simulink model "B100A_Inlet"  (R2024a)
settings: Solver=VariableStepAuto  StartTime=0.0  StopTime=10.0  RelTol=1e-3
undefined symbols (not defined in the file): CCS1, CCS2, GB, T, Type1, Type2
libraries: simulink x2
settings Model: DataDictionary=EVSE_Root_dict.sldd  Creator=jh2beauty  LastModifiedBy=jh2beauty

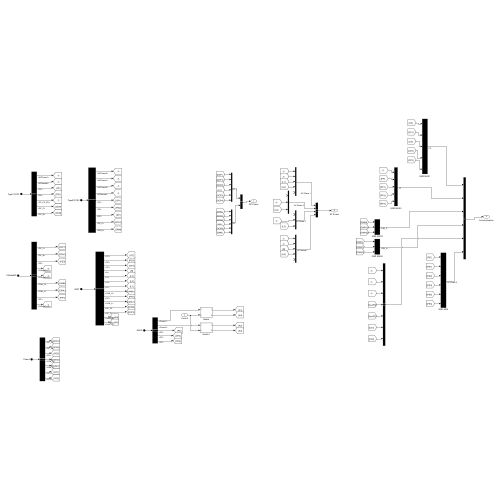
[thumbnail: Simulink's stored preview of the top-level diagram]
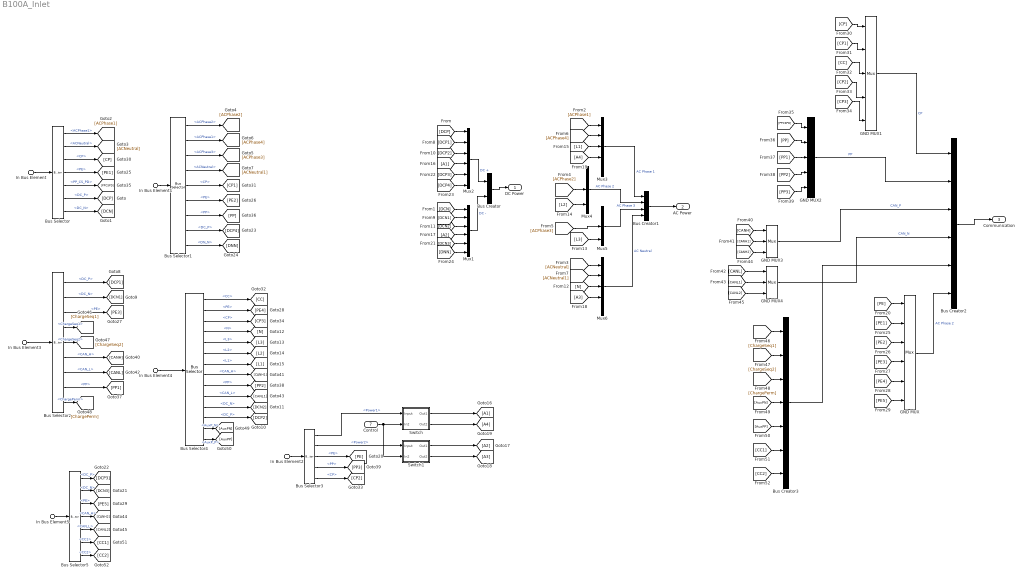
== system B100A_Inlet ==
  In Bus Element : Inport  PortName=Type1/CCS1
  In Bus Element1 : Inport  Port=2  PortName=Type2/CCS2
  In Bus Element2 : Inport  Port=3  PortName=NACS
  In Bus Element3 : Inport  Port=4  PortName=CHAdeMO
  In Bus Element4 : Inport  Port=5  PortName=GB/T
  In Bus Element5 : Inport  Port=6  PortName=ChaoJi
  Control : Inport  Port=7
  Bus Creator : BusCreator  Inputs=2
  Bus Creator1 : BusCreator  Inputs=4
  Bus Creator2 : BusCreator  Inputs=6
  Bus Creator3 : BusCreator  Inputs=7
  Bus Selector : BusSelector  OutputSignals=ACPhase1,ACNeutral,CP,PE,PP_CS_PD,DC_P,DC_N
  Bus Selector1 : BusSelector  OutputSignals=ACPhase2,ACPhase1,ACPhase3,ACNeutral,CP,PE,PP,DC_P,DN_N
  Bus Selector2 : BusSelector  OutputSignals=DC_P,DC_N,PE,ChargeSeq1,ChargeSeq2,CAN_H,CAN_L,PP,ChargePerm
  Bus Selector3 : BusSelector  OutputSignals=Power1,Power2,PE,PP,CP
  Bus Selector4 : BusSelector  OutputSignals=CC,PE,CP,N,L3,L2,L1,CAN_H,PP,CAN_L,DC_N,DC_P,AuxP_N,AuxP_P
  Bus Selector5 : BusSelector  OutputSignals=DC_P,DC_N,PE,CAN_H,CAN_L,CC1,CC2
  GND MUX : Mux  Inputs=6
  GND MUX1 : Mux  Inputs=5
  GND MUX2 : Mux  Inputs=5
  GND MUX3 : Mux  Inputs=3
  GND MUX4 : Mux  Inputs=3
  Mux1 : Mux  Inputs=6
  Mux2 : Mux  Inputs=6
  Mux3 : Mux  Inputs=5
  Mux4 : Mux  Inputs=3
  Mux5 : Mux  Inputs=3
  Mux6 : Mux  Inputs=5
  Switch : Subsystem
  Switch1 : Subsystem
  DC Power : Outport
  AC Power : Outport  Port=2
  Communication : Outport  Port=3
  wires:
  In Bus Element/1 -> Bus Selector/1
  In Bus Element1/1 -> Bus Selector1/1
  Bus Creator/1 -> DC Power/1
  Bus Creator1/1 -> AC Power/1
  Bus Creator2/1 -> Communication/1
  Mux2/1 -> Bus Creator/1  "DC +"
  Mux1/1 -> Bus Creator/2  "DC -"
  Mux3/1 -> Bus Creator1/1  "AC Phase 1"
  Mux4/1 -> Bus Creator1/2  "AC Phase 2"
  Mux5/1 -> Bus Creator1/3  "AC Phase 3"
  Mux6/1 -> Bus Creator1/4  "AC Neutral"
  In Bus Element3/1 -> Bus Selector2/1
  In Bus Element2/1 -> Bus Selector3/1
  Bus Selector/6 -> [DCP]  "<DC_P>"
  [DCP] -> Mux2/1
  Bus Selector/7 -> [DCN]  "<DC_N>"
  [DCN] -> Mux1/1
  Bus Selector/1 -> [ACPhase1]  "<ACPhase1>"
  [ACPhase1] -> Mux3/1
  Bus Selector/2 -> [ACNeutral]  "<ACNeutral>"
  [ACNeutral] -> Mux6/1
  Bus Selector1/1 -> [ACPhase2]  "<ACPhase2>"
  [ACPhase2] -> Mux4/2
  Bus Selector1/3 -> [ACPhase3]  "<ACPhase3>"
  [ACPhase3] -> Mux5/2
  Bus Selector1/2 -> [ACPhase4]  "<ACPhase1>"
  [ACPhase4] -> Mux3/2
  Bus Selector1/4 -> [ACNeutral1]  "<ACNeutral>"
  [ACNeutral1] -> Mux6/2
  In Bus Element4/1 -> Bus Selector4/1
  In Bus Element5/1 -> Bus Selector5/1
  Bus Selector3/1 -> Switch/1(Input)  "<Power1>"
  Bus Selector3/2 -> Switch1/1(Input)  "<Power2>"
  Bus Selector2/1 -> [DCP1]  "<DC_P>"
  [DCP1] -> Mux2/2
  Bus Selector2/2 -> [DCN1]  "<DC_N>"
  [DCN1] -> Mux1/2
  Bus Selector4/12 -> [DCP2]  "<DC_P>"
  [DCP2] -> Mux2/3
  Bus Selector4/11 -> [DCN2]  "<DC_N>"
  [DCN2] -> Mux1/3
  Bus Selector4/4 -> [N]  "<N>"
  [N] -> Mux6/3
  Bus Selector4/5 -> [L3]  "<L3>"
  [L3] -> Mux5/3
  Bus Selector4/6 -> [L2]  "<L2>"
  [L2] -> Mux4/3
  Bus Selector4/7 -> [L1]  "<L1>"
  [L1] -> Mux3/3
  Switch/1(Out1) -> [A1]
  [A1] -> Mux2/4
  Switch1/1(Out1) -> [A2]
  [A2] -> Mux1/4
  Switch1/2(Out2) -> [A3]
  [A3] -> Mux6/4
  Switch/2(Out2) -> [A4]
  [A4] -> Mux3/4
  Control/1 -> Switch1/2(In2), Switch/2(In2)
  Bus Selector3/3 -> [PE]  "<PE>"
  [PE] -> GND MUX/1
  Bus Selector5/2 -> [DCN3]  "<DC_N>"
  [DCN3] -> Mux1/5
  Bus Selector5/1 -> [DCP3]  "<DC_P>"
  [DCP3] -> Mux2/5
  Bus Selector1/8 -> [DCP4]  "<DC_P>"
  [DCP4] -> Mux2/6
  Bus Selector1/9 -> [DNN]  "<DN_N>"
  [DNN] -> Mux1/6
  Bus Selector/4 -> [PE1]  "<PE>"
  [PE1] -> GND MUX/2
  Bus Selector1/6 -> [PE2]  "<PE>"
  [PE2] -> GND MUX/3
  Bus Selector2/3 -> [PE3]  "<PE>"
  [PE3] -> GND MUX/4
  Bus Selector4/2 -> [PE4]  "<PE>"
  [PE4] -> GND MUX/5
  Bus Selector5/3 -> [PE5]  "<PE>"
  [PE5] -> GND MUX/6
  Bus Selector/3 -> [CP]  "<CP>"
  [CP] -> GND MUX1/1
  Bus Selector1/5 -> [CP1]  "<CP>"
  [CP1] -> GND MUX1/2
  Bus Selector4/1 -> [CC]  "<CC>"
  [CC] -> GND MUX1/3
  Bus Selector3/5 -> [CP2]  "<CP>"
  [CP2] -> GND MUX1/4
  Bus Selector4/3 -> [CP3]  "<CP>"
  [CP3] -> GND MUX1/5
  Bus Selector/5 -> [PPCSPD]  "<PP_CS_PD>"
  [PPCSPD] -> GND MUX2/1
  Bus Selector1/7 -> [PP]  "<PP>"
  [PP] -> GND MUX2/2
  Bus Selector2/8 -> [PP1]  "<PP>"
  [PP1] -> GND MUX2/3
  Bus Selector4/9 -> [PP2]  "<PP>"
  [PP2] -> GND MUX2/4
  Bus Selector3/4 -> [PP3]  "<PP>"
  [PP3] -> GND MUX2/5
  GND MUX1/1 -> Bus Creator2/1  "CP"
  GND MUX2/1 -> Bus Creator2/2  "PP"
  Bus Selector2/6 -> [CANH]  "<CAN_H>"
  [CANH] -> GND MUX3/1
  Bus Selector4/8 -> [CANH1]  "<CAN_H>"
  [CANH1] -> GND MUX3/2
  Bus Selector2/7 -> [CANL]  "<CAN_L>"
  [CANL] -> GND MUX4/1
  Bus Selector4/10 -> [CANL1]  "<CAN_L>"
  [CANL1] -> GND MUX4/2
  GND MUX3/1 -> Bus Creator2/3  "CAN_P"
  GND MUX4/1 -> Bus Creator2/4  "CAN_N"
  Bus Selector5/4 -> [CANH2]  "<CAN_H>"
  [CANH2] -> GND MUX3/3
  Bus Selector5/5 -> [CANL2]  "<CAN_L>"
  [CANL2] -> GND MUX4/3
  GND MUX/1 -> Bus Creator2/6  "AC Phase 2"
  Bus Creator3/1 -> Bus Creator2/5
  Bus Selector2/4 -> [ChargeSeq1]  "<ChargeSeq1>"
  [ChargeSeq1] -> Bus Creator3/1
  Bus Selector2/5 -> [ChargeSeq2]  "<ChargeSeq2>"
  [ChargeSeq2] -> Bus Creator3/2
  Bus Selector2/9 -> [ChargePerm]  "<ChargePerm>"
  [ChargePerm] -> Bus Creator3/3
  Bus Selector4/13 -> [AuxPN]  "<AuxP_N>"
  [AuxPN] -> Bus Creator3/4
  Bus Selector4/14 -> [AuxPP]  "<AuxP_P>"
  [AuxPP] -> Bus Creator3/5
  Bus Selector5/6 -> [CC1]  "<CC1>"
  [CC1] -> Bus Creator3/6
  Bus Selector5/7 -> [CC2]  "<CC2>"
  [CC2] -> Bus Creator3/7

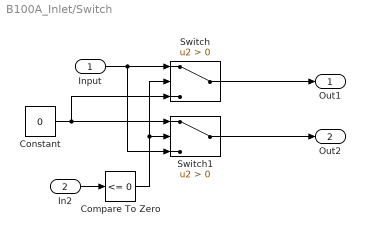
== system B100A_Inlet/Switch ==
  Input : Inport
  In2 : Inport  Port=2
  Compare To Zero : simulink/Logic and Bit Operations/Compare To Zero  relop=<=  OutDataTypeStr=boolean
  Constant : Constant  Value=0
  Switch : Switch  Criteria=u2 > Threshold  SaturateOnIntegerOverflow=off  InputSameDT=off
  Switch1 : Switch  Criteria=u2 > Threshold  SaturateOnIntegerOverflow=off  InputSameDT=off
  Out1 : Outport
  Out2 : Outport  Port=2
  wires:
  Input/1 -> Switch1/3, Switch/1
  Switch/1 -> Out1/1
  Switch1/1 -> Out2/1
  Constant/1 -> Switch1/1, Switch/3
  In2/1 -> Compare To Zero/1
  Compare To Zero/1 -> Switch/2, Switch1/2

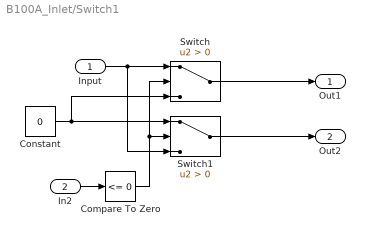
== system B100A_Inlet/Switch1 ==
  Input : Inport
  In2 : Inport  Port=2
  Compare To Zero : simulink/Logic and Bit Operations/Compare To Zero  relop=<=  OutDataTypeStr=boolean
  Constant : Constant  Value=0
  Switch : Switch  Criteria=u2 > Threshold  SaturateOnIntegerOverflow=off  InputSameDT=off
  Switch1 : Switch  Criteria=u2 > Threshold  SaturateOnIntegerOverflow=off  InputSameDT=off
  Out1 : Outport
  Out2 : Outport  Port=2
  wires:
  Input/1 -> Switch1/3, Switch/1
  Switch/1 -> Out1/1
  Switch1/1 -> Out2/1
  Constant/1 -> Switch1/1, Switch/3
  In2/1 -> Compare To Zero/1
  Compare To Zero/1 -> Switch/2, Switch1/2
